simulink model "AMCLIB_FWSpeedLoop_BAM_FLT"  (Simulink 8.3)
settings: Solver=ode45  StartTime=0.0  StopTime=10.0  RelTol=1e-3
undefined symbols (not defined in the file): fltIntegGainFW, fltIntegGainQ, fltLambdaFW, fltLambdaW, fltPropGainFW, fltPropGainQ, fltRampDown, fltRampUp, fltUmaxDivImax
settings Model: Creator=B37097  LastModifiedBy=B37097
settings DataIOCC: SignalLoggingSaveFormat=Dataset
settings DebuggingCC: UnderspecifiedInitializationDetection=Simplified  StateNameClashWarn=none
settings GRTTargetCC: CombineOutputUpdateFcns=on  GRTInterface=off

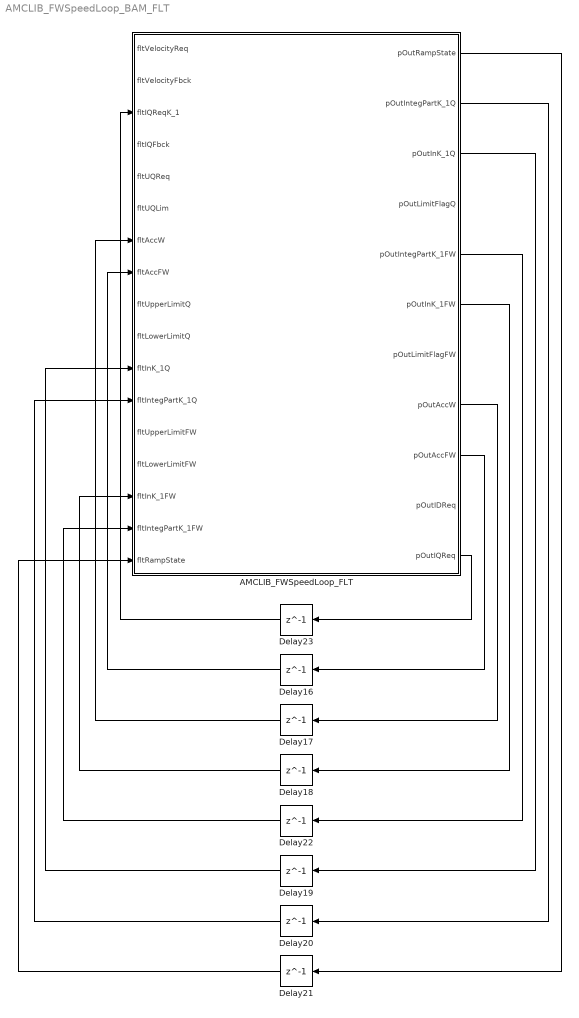
== system AMCLIB_FWSpeedLoop_BAM_FLT ==
  AMCLIB_FWSpeedLoop_FLT : Subsystem  mask(AMCLIB_FWSpeedLoop_FLT){fltLambdaW=fltLambdaW, fltLambdaFW=fltLambdaFW, fltPropGainQ=fltPropGainQ, fltIntegGainQ=fltIntegGainQ, fltPropGainFW=fltPropGainFW, fltIntegGainFW=fltIntegGainFW, fltRampUp=fltRampUp, fltRampDown=fltRampDown, fltUmaxDivImax=fltUmaxDivImax}
      mask help: Bit accurate model of the speed loop algorithm with field weakening capability. All parameters as well as input and output values are in single precision floating data format.
      mask init:
      | pos = get_param(gcb, 'Position');width = pos(3) - pos(1); height = pos(4) - pos(2);tX=width/2;tY=height*0.9;
      mask Display: color('black');port_label('input',1,'fltVelocityReq');port_label('input',2,'fltVelocityFbck');port_label('input',3,'fltIQReqK_1');port_label('input',4,'fltIQFbck');port_label('input',5,'fltUQReq');port_label('input',6,'fltUQLim');port_label('input',7,'fltAccW');port_label('input',8,'fltAccFW');port_label('input',9,'fltUpperLimitQ');port_label('input',10,'fltLowerLimitQ');port_label('input',11,'fltInK_1Q');port_label('input',12,'fltIntegPartK_1Q');port_label('input',13,'fltUpperLimitFW');port_label('input',14,'fltLowerLimitFW');port_label('input',15,'fltInK_1FW');port_label('input',16,'fltIntegPartK_1FW');port_label('input',17,'fltRampState');port_label('output',1,'pOutRampState');port_label('output',2,'pOutIntegPartK_1Q');port_label('output',3,'pOutInK_1Q');port_label('output',4,'pOutLimitFlagQ');port_label('output',5,'pOutIntegPartK_1FW');port_label('output',6,'pOutInK_1FW');port_label('output',7,'pOutLimitFlagFW');port_label('output',8,'pOutAccW');port_label('output',9,'pOutAccFW');port_label('output',10,'pOutIDReq');port_label('output',11,'pOutIQReq');color('black');disp('AMCLIB_FWSpeedLoop_FLT');color('blue');text(tX,tY, 'BAM', 'horizontalAlignment', 'center');
  Delay{16..23} (8 alike) : Delay  DelayLength=1  InitialCondition=0
  wires:
  AMCLIB_FWSpeedLoop_FLT/11(pOutIQReq) -> Delay23/1
  Delay23/1 -> AMCLIB_FWSpeedLoop_FLT/3(fltIQReqK_1)
  AMCLIB_FWSpeedLoop_FLT/9(pOutAccFW) -> Delay16/1
  Delay16/1 -> AMCLIB_FWSpeedLoop_FLT/8(fltAccFW)
  AMCLIB_FWSpeedLoop_FLT/8(pOutAccW) -> Delay17/1
  Delay17/1 -> AMCLIB_FWSpeedLoop_FLT/7(fltAccW)
  AMCLIB_FWSpeedLoop_FLT/6(pOutInK_1FW) -> Delay18/1
  Delay18/1 -> AMCLIB_FWSpeedLoop_FLT/15(fltInK_1FW)
  AMCLIB_FWSpeedLoop_FLT/5(pOutIntegPartK_1FW) -> Delay22/1
  Delay22/1 -> AMCLIB_FWSpeedLoop_FLT/16(fltIntegPartK_1FW)
  AMCLIB_FWSpeedLoop_FLT/3(pOutInK_1Q) -> Delay19/1
  Delay19/1 -> AMCLIB_FWSpeedLoop_FLT/11(fltInK_1Q)
  AMCLIB_FWSpeedLoop_FLT/2(pOutIntegPartK_1Q) -> Delay20/1
  Delay20/1 -> AMCLIB_FWSpeedLoop_FLT/12(fltIntegPartK_1Q)
  AMCLIB_FWSpeedLoop_FLT/1(pOutRampState) -> Delay21/1
  Delay21/1 -> AMCLIB_FWSpeedLoop_FLT/17(fltRampState)

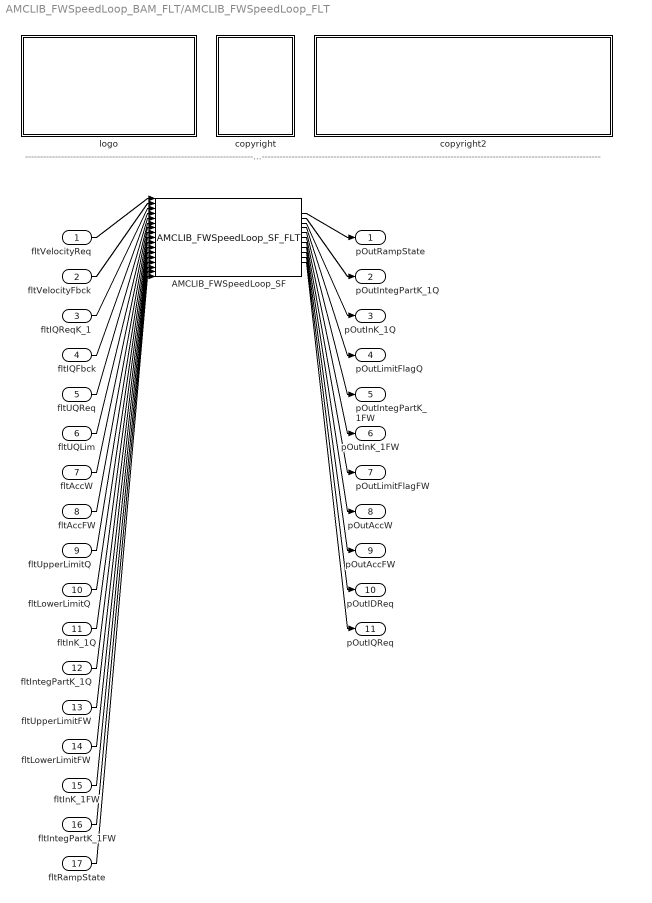
== system AMCLIB_FWSpeedLoop_BAM_FLT/AMCLIB_FWSpeedLoop_FLT ==
  note: ---------------------------------------------------------------------------------------------------------------------------------------------------------------------------------------------------
  fltVelocityReq : Inport
  fltVelocityFbck : Inport  Port=2
  fltIQReqK_1 : Inport  Port=3
  fltIQFbck : Inport  Port=4
  fltUQReq : Inport  Port=5
  fltUQLim : Inport  Port=6
  fltAccW : Inport  Port=7
  fltAccFW : Inport  Port=8
  fltUpperLimitQ : Inport  Port=9
  fltLowerLimitQ : Inport  Port=10
  fltInK_1Q : Inport  Port=11
  fltIntegPartK_1Q : Inport  Port=12
  fltUpperLimitFW : Inport  Port=13
  fltLowerLimitFW : Inport  Port=14
  fltInK_1FW : Inport  Port=15
  fltIntegPartK_1FW : Inport  Port=16
  fltRampState : Inport  Port=17
  AMCLIB_FWSpeedLoop_SF : S-Function  FunctionName=AMCLIB_FWSpeedLoop_SF_FLT  Parameters=fltLambdaW,fltLambdaFW,fltPropGainQ,fltIntegGainQ,fltPropGainFW,fltIntegGainFW,fltRampUp,fltRampDown,fltUmaxDivImax  EnableBusSupport=off
  copyright : Subsystem
      mask Display: text(10,90,'FILE:');text(10,75,'DESRIPTION:');text(10,60,'COPYRIGHT:');text(10,45,'VERSION:');text(10,30,'DATE:')
  copyright2 : Subsystem
      mask Display: text(10,90,'AMCLIB_FWSpeedLoop_BAM_FLT.mdl');text(10,75,'Speed Loop with Field Weakening.');text(10,60,'NXP');text(10,45,'1.0');text(10,30,'14-Sep-2017');
  logo : Subsystem
      mask Display: image(imread('logo.jpg'))
  pOutRampState : Outport
  pOutIntegPartK_1Q : Outport  Port=2
  pOutInK_1Q : Outport  Port=3
  pOutLimitFlagQ : Outport  Port=4
  pOutIntegPartK_1FW : Outport  Port=5
  pOutInK_1FW : Outport  Port=6
  pOutLimitFlagFW : Outport  Port=7
  pOutAccW : Outport  Port=8
  pOutAccFW : Outport  Port=9
  pOutIDReq : Outport  Port=10
  pOutIQReq : Outport  Port=11
  wires:
  fltVelocityReq/1 -> AMCLIB_FWSpeedLoop_SF/1
  fltVelocityFbck/1 -> AMCLIB_FWSpeedLoop_SF/2
  fltIQReqK_1/1 -> AMCLIB_FWSpeedLoop_SF/3
  fltIQFbck/1 -> AMCLIB_FWSpeedLoop_SF/4
  fltUQReq/1 -> AMCLIB_FWSpeedLoop_SF/5
  fltUQLim/1 -> AMCLIB_FWSpeedLoop_SF/6
  fltAccW/1 -> AMCLIB_FWSpeedLoop_SF/7
  fltAccFW/1 -> AMCLIB_FWSpeedLoop_SF/8
  fltUpperLimitQ/1 -> AMCLIB_FWSpeedLoop_SF/9
  fltLowerLimitQ/1 -> AMCLIB_FWSpeedLoop_SF/10
  fltInK_1Q/1 -> AMCLIB_FWSpeedLoop_SF/11
  fltIntegPartK_1Q/1 -> AMCLIB_FWSpeedLoop_SF/12
  fltUpperLimitFW/1 -> AMCLIB_FWSpeedLoop_SF/13
  fltLowerLimitFW/1 -> AMCLIB_FWSpeedLoop_SF/14
  fltInK_1FW/1 -> AMCLIB_FWSpeedLoop_SF/15
  fltIntegPartK_1FW/1 -> AMCLIB_FWSpeedLoop_SF/16
  fltRampState/1 -> AMCLIB_FWSpeedLoop_SF/17
  AMCLIB_FWSpeedLoop_SF/1 -> pOutRampState/1
  AMCLIB_FWSpeedLoop_SF/2 -> pOutIntegPartK_1Q/1
  AMCLIB_FWSpeedLoop_SF/3 -> pOutInK_1Q/1
  AMCLIB_FWSpeedLoop_SF/4 -> pOutLimitFlagQ/1
  AMCLIB_FWSpeedLoop_SF/5 -> pOutIntegPartK_1FW/1
  AMCLIB_FWSpeedLoop_SF/6 -> pOutInK_1FW/1
  AMCLIB_FWSpeedLoop_SF/7 -> pOutLimitFlagFW/1
  AMCLIB_FWSpeedLoop_SF/8 -> pOutAccW/1
  AMCLIB_FWSpeedLoop_SF/9 -> pOutAccFW/1
  AMCLIB_FWSpeedLoop_SF/10 -> pOutIDReq/1
  AMCLIB_FWSpeedLoop_SF/11 -> pOutIQReq/1

== system AMCLIB_FWSpeedLoop_BAM_FLT/AMCLIB_FWSpeedLoop_FLT/copyright ==

== system AMCLIB_FWSpeedLoop_BAM_FLT/AMCLIB_FWSpeedLoop_FLT/copyright2 ==

== system AMCLIB_FWSpeedLoop_BAM_FLT/AMCLIB_FWSpeedLoop_FLT/logo ==
